simulink model "TrajectoryPlanningEmulation"  (R2018b)
settings: configuration reference "Active" (kept outside this file)
model workspace (MAT data in the model file):
  Raceline.s_m = [0 0 0 0 0 0 0 0 0 0 0 0 ... (5000 elements, 5000x1)]
  Raceline.x_m = [0 0 0 0 0 0 0 0 0 0 0 0 ... (5000 elements, 5000x1)]
  Raceline.y_m = [0 0 0 0 0 0 0 0 0 0 0 0 ... (5000 elements, 5000x1)]
  Raceline.psi_rad = [0 0 0 0 0 0 0 0 0 0 0 0 ... (5000 elements, 5000x1)]
  Raceline.kappa_radpm = [0 0 0 0 0 0 0 0 0 0 0 0 ... (5000 elements, 5000x1)]
  Raceline.vx_mps = [0 0 0 0 0 0 0 0 0 0 0 0 ... (5000 elements, 5000x1)]
  Raceline.ax_mps2 = [0 0 0 0 0 0 0 0 0 0 0 0 ... (5000 elements, 5000x1)]
  Raceline.delta_rad = [0 0 0 0 0 0 0 0 0 0 0 0 ... (5000 elements, 5000x1)]
  Raceline.F_N = [0 0 0 0 0 0 0 0 0 0 0 0 ... (5000 elements, 5000x1)]
  Raceline.ValidPointCnt = 0
  Raceline.s_m_end = 0
undefined symbols (not defined in the file): ActivateTP_PX2, P_PX2_VirtualDelay_s, tS, tSSlow, TUMHealthStatus, TUMStrategyState, TUMVehicleState
settings Model: DataDictionary=TrajectoryPlanningEmulation.sldd  ParameterArgumentNames=Raceline  OrderedModelArguments=off  Creator=wischnewski  LastModifiedBy=ge34qer

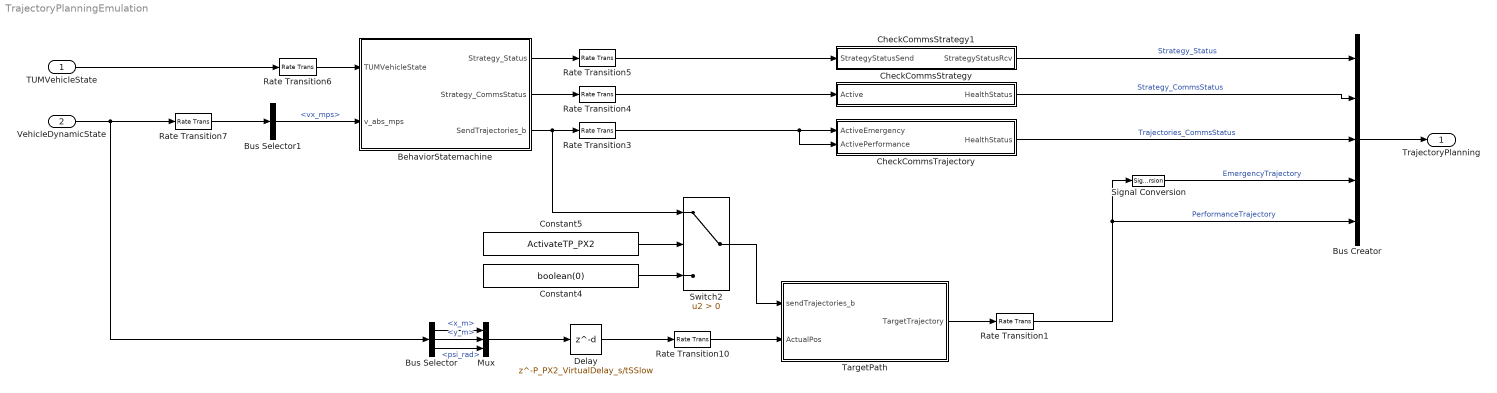
== system TrajectoryPlanningEmulation ==
  TUMVehicleState : Inport  OutDataTypeStr=Enum: TUMVehicleState  SampleTime=tS
  VehicleDynamicState : Inport  Port=2  OutDataTypeStr=Bus: VehicleDynamicState  SampleTime=tS
  BehaviorStatemachine : Subsystem  TreatAsAtomicUnit=on  SystemSampleTime=tSSlow
  Bus Creator : BusCreator  Inputs=5
  Bus Selector : BusSelector  OutputSignals=Pos.x_m,Pos.y_m,Pos.psi_rad
  Bus Selector1 : BusSelector  OutputSignals=vx_mps
  CheckCommsStrategy : Subsystem
  CheckCommsStrategy1 : Subsystem
  CheckCommsTrajectory : Subsystem
  Constant4 : Constant  Value=boolean(0)
  Constant5 : Constant  Value=ActivateTP_PX2
  Delay : Delay  DelayLength=P_PX2_VirtualDelay_s/tSSlow
  Mux : Mux  Inputs=3
  Rate Transition{1,3..4,7,10} (5 alike) : RateTransition
  Rate Transition5 : RateTransition  InitialCondition=TUMStrategyState.S_OFF
  Rate Transition6 : RateTransition  InitialCondition=TUMVehicleState.OFF
  Signal Conversion : SignalConversion  OverrideOpt=off
  Switch2 : Switch  Criteria=u2 > Threshold
  TargetPath : Subsystem  TreatAsAtomicUnit=on  SystemSampleTime=tSSlow
  TrajectoryPlanning : Outport  OutDataTypeStr=Bus: TrajectoryPlanning  SampleTime=tS  BusOutputAsStruct=on
  wires:
  Bus Creator/1 -> TrajectoryPlanning/1
  Signal Conversion/1 -> Bus Creator/4  "EmergencyTrajectory"
  VehicleDynamicState/1 -> Bus Selector/1, Rate Transition7/1
  Delay/1 -> Rate Transition10/1
  BehaviorStatemachine/1(Strategy_Status) -> Rate Transition5/1
  BehaviorStatemachine/2(Strategy_CommsStatus) -> Rate Transition4/1
  CheckCommsTrajectory/1(HealthStatus) -> Bus Creator/3  "Trajectories_CommsStatus"
  Rate Transition1/1 -> Signal Conversion/1, Bus Creator/5  "PerformanceTrajectory"
  TargetPath/1(TargetTrajectory) -> Rate Transition1/1
  CheckCommsStrategy/1(HealthStatus) -> Bus Creator/2  "Strategy_CommsStatus"
  CheckCommsStrategy1/1(StrategyStatusRcv) -> Bus Creator/1  "Strategy_Status"
  Rate Transition6/1 -> BehaviorStatemachine/1(TUMVehicleState)
  Rate Transition7/1 -> Bus Selector1/1
  Rate Transition4/1 -> CheckCommsStrategy/1(Active)
  Rate Transition5/1 -> CheckCommsStrategy1/1(StrategyStatusSend)
  Constant5/1 -> Switch2/2
  BehaviorStatemachine/3(SendTrajectories_b) -> Switch2/1, Rate Transition3/1
  Constant4/1 -> Switch2/3
  Rate Transition3/1 -> CheckCommsTrajectory/2(ActivePerformance), CheckCommsTrajectory/1(ActiveEmergency)
  Switch2/1 -> TargetPath/1(sendTrajectories_b)
  Bus Selector1/1 -> BehaviorStatemachine/2(v_abs_mps)  "<vx_mps>"
  Rate Transition10/1 -> TargetPath/2(ActualPos)
  Bus Selector/2 -> Mux/2  "<y_m>"
  Bus Selector/1 -> Mux/1  "<x_m>"
  Bus Selector/3 -> Mux/3  "<psi_rad>"
  Mux/1 -> Delay/1
  TUMVehicleState/1 -> Rate Transition6/1

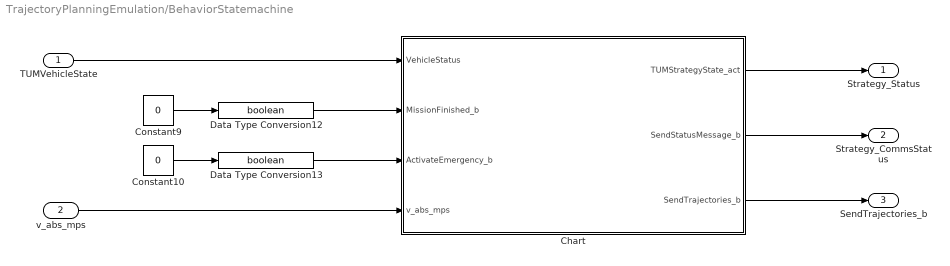
== system TrajectoryPlanningEmulation/BehaviorStatemachine ==
  TUMVehicleState : Inport  OutDataTypeStr=Enum: TUMVehicleState
  v_abs_mps : Inport  Port=2
  Chart : Stateflow chart  TreatAsAtomicUnit=on
  Constant10 : Constant  Value=0
  Constant9 : Constant  Value=0
  Data Type Conversion12 : DataTypeConversion  OutDataTypeStr=boolean
  Data Type Conversion13 : DataTypeConversion  OutDataTypeStr=boolean
  Strategy_Status : Outport
  Strategy_CommsStatus : Outport  Port=2
  SendTrajectories_b : Outport  Port=3
  wires:
  Constant10/1 -> Data Type Conversion13/1
  Data Type Conversion13/1 -> Chart/3(ActivateEmergency_b)
  v_abs_mps/1 -> Chart/4(v_abs_mps)
  Chart/3(SendTrajectories_b) -> SendTrajectories_b/1
  TUMVehicleState/1 -> Chart/1(VehicleStatus)
  Data Type Conversion12/1 -> Chart/2(MissionFinished_b)
  Constant9/1 -> Data Type Conversion12/1
  Chart/2(SendStatusMessage_b) -> Strategy_CommsStatus/1
  Chart/1(TUMStrategyState_act) -> Strategy_Status/1

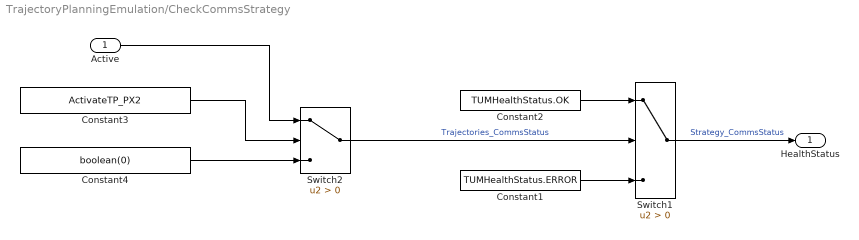
== system TrajectoryPlanningEmulation/CheckCommsStrategy ==
  Active : Inport
  Constant1 : Constant  Value=TUMHealthStatus.ERROR  OutDataTypeStr=Enum: TUMHealthStatus
  Constant2 : Constant  Value=TUMHealthStatus.OK  OutDataTypeStr=Enum: TUMHealthStatus
  Constant3 : Constant  Value=ActivateTP_PX2
  Constant4 : Constant  Value=boolean(0)
  Switch1 : Switch  Criteria=u2 > Threshold
  Switch2 : Switch  Criteria=u2 > Threshold
  HealthStatus : Outport
  wires:
  Constant2/1 -> Switch1/1
  Switch1/1 -> HealthStatus/1  "Strategy_CommsStatus"
  Constant1/1 -> Switch1/3
  Constant3/1 -> Switch2/2
  Active/1 -> Switch2/1
  Constant4/1 -> Switch2/3
  Switch2/1 -> Switch1/2  "Trajectories_CommsStatus"

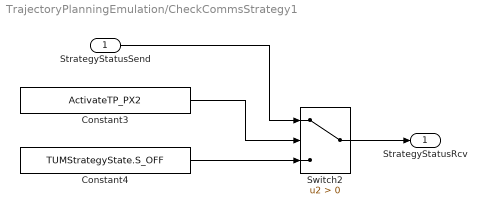
== system TrajectoryPlanningEmulation/CheckCommsStrategy1 ==
  StrategyStatusSend : Inport
  Constant3 : Constant  Value=ActivateTP_PX2
  Constant4 : Constant  Value=TUMStrategyState.S_OFF
  Switch2 : Switch  Criteria=u2 > Threshold
  StrategyStatusRcv : Outport
  wires:
  Constant3/1 -> Switch2/2
  StrategyStatusSend/1 -> Switch2/1
  Constant4/1 -> Switch2/3
  Switch2/1 -> StrategyStatusRcv/1

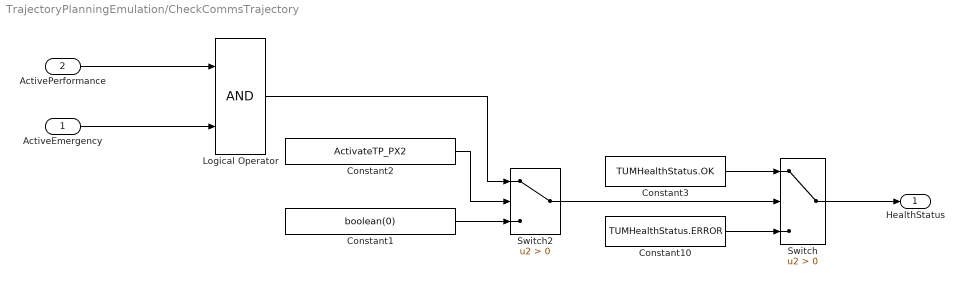
== system TrajectoryPlanningEmulation/CheckCommsTrajectory ==
  ActiveEmergency : Inport
  ActivePerformance : Inport  Port=2
  Constant1 : Constant  Value=boolean(0)
  Constant10 : Constant  Value=TUMHealthStatus.ERROR  OutDataTypeStr=Enum: TUMHealthStatus
  Constant2 : Constant  Value=ActivateTP_PX2
  Constant3 : Constant  Value=TUMHealthStatus.OK  OutDataTypeStr=Enum: TUMHealthStatus
  Logical Operator : Logic  AllPortsSameDT=off  OutDataTypeStr=boolean
  Switch : Switch  Criteria=u2 > Threshold
  Switch2 : Switch  Criteria=u2 > Threshold
  HealthStatus : Outport
  wires:
  Constant10/1 -> Switch/3
  Switch2/1 -> Switch/2
  Constant3/1 -> Switch/1
  Switch/1 -> HealthStatus/1
  Constant2/1 -> Switch2/2
  Logical Operator/1 -> Switch2/1
  Constant1/1 -> Switch2/3
  ActivePerformance/1 -> Logical Operator/1
  ActiveEmergency/1 -> Logical Operator/2

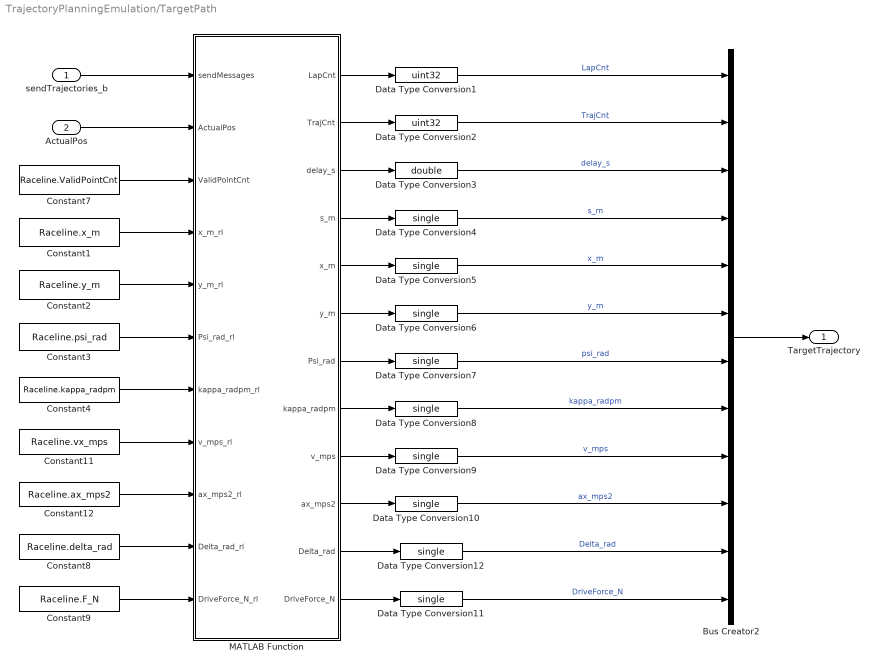
== system TrajectoryPlanningEmulation/TargetPath ==
  sendTrajectories_b : Inport
  ActualPos : Inport  Port=2  PortDimensions=3
  Bus Creator2 : BusCreator  Inputs=12  OutDataTypeStr=Bus: Trajectory
      settings: InheritFromInputs=off
  Constant1 : Constant  Value=Raceline.x_m
  Constant11 : Constant  Value=Raceline.vx_mps
  Constant12 : Constant  Value=Raceline.ax_mps2
  Constant2 : Constant  Value=Raceline.y_m
  Constant3 : Constant  Value=Raceline.psi_rad
  Constant4 : Constant  Value=Raceline.kappa_radpm
  Constant7 : Constant  Value=Raceline.ValidPointCnt
  Constant8 : Constant  Value=Raceline.delta_rad
  Constant9 : Constant  Value=Raceline.F_N
  Data Type Conversion1 : DataTypeConversion  OutDataTypeStr=uint32
  Data Type Conversion{4..12} (9 alike) : DataTypeConversion  OutDataTypeStr=single
  Data Type Conversion2 : DataTypeConversion  OutDataTypeStr=uint32
  Data Type Conversion3 : DataTypeConversion  OutDataTypeStr=double
  MATLAB Function : MATLAB Function  TreatAsAtomicUnit=on
  TargetTrajectory : Outport  OutDataTypeStr=Bus: Trajectory
  wires:
  MATLAB Function/1(LapCnt) -> Data Type Conversion1/1
  Data Type Conversion4/1 -> Bus Creator2/4  "s_m"
  Data Type Conversion5/1 -> Bus Creator2/5  "x_m"
  Data Type Conversion6/1 -> Bus Creator2/6  "y_m"
  Data Type Conversion7/1 -> Bus Creator2/7  "psi_rad"
  Data Type Conversion8/1 -> Bus Creator2/8  "kappa_radpm"
  Data Type Conversion9/1 -> Bus Creator2/9  "v_mps"
  Data Type Conversion10/1 -> Bus Creator2/10  "ax_mps2"
  MATLAB Function/4(s_m) -> Data Type Conversion4/1
  MATLAB Function/5(x_m) -> Data Type Conversion5/1
  MATLAB Function/6(y_m) -> Data Type Conversion6/1
  MATLAB Function/7(Psi_rad) -> Data Type Conversion7/1
  MATLAB Function/8(kappa_radpm) -> Data Type Conversion8/1
  MATLAB Function/9(v_mps) -> Data Type Conversion9/1
  MATLAB Function/10(ax_mps2) -> Data Type Conversion10/1
  Data Type Conversion1/1 -> Bus Creator2/1  "LapCnt"
  Data Type Conversion2/1 -> Bus Creator2/2  "TrajCnt"
  Constant1/1 -> MATLAB Function/4(x_m_rl)
  Constant2/1 -> MATLAB Function/5(y_m_rl)
  Constant3/1 -> MATLAB Function/6(Psi_rad_rl)
  Constant4/1 -> MATLAB Function/7(kappa_radpm_rl)
  MATLAB Function/2(TrajCnt) -> Data Type Conversion2/1
  Constant7/1 -> MATLAB Function/3(ValidPointCnt)
  Bus Creator2/1 -> TargetTrajectory/1
  ActualPos/1 -> MATLAB Function/2(ActualPos)
  Data Type Conversion3/1 -> Bus Creator2/3  "delay_s"
  sendTrajectories_b/1 -> MATLAB Function/1(sendMessages)
  MATLAB Function/3(delay_s) -> Data Type Conversion3/1
  Data Type Conversion12/1 -> Bus Creator2/11  "Delta_rad"
  Data Type Conversion11/1 -> Bus Creator2/12  "DriveForce_N"
  MATLAB Function/11(Delta_rad) -> Data Type Conversion12/1
  MATLAB Function/12(DriveForce_N) -> Data Type Conversion11/1
  Constant8/1 -> MATLAB Function/10(Delta_rad_rl)
  Constant9/1 -> MATLAB Function/11(DriveForce_N_rl)
  Constant11/1 -> MATLAB Function/8(v_mps_rl)
  Constant12/1 -> MATLAB Function/9(ax_mps2_rl)

== matlab function TrajectoryPlanningEmulation/TargetPath/MATLAB Function ==
  data: sendMessages input; ActualPos input; ValidPointCnt input; LapCnt output size=1; x_m_rl input; y_m_rl input; Psi_rad_rl input; kappa_radpm_rl input; v_mps_rl input; ax_mps2_rl input; TrajCnt output size=1; delay_s output; s_m output size=50; x_m output size=50; y_m output size=50; Psi_rad output size=50; kappa_radpm output size=50; v_mps output size=50; ax_mps2 output size=50; Delta_rad output; DriveForce_N output; Delta_rad_rl input; DriveForce_N_rl input
function [LapCnt, TrajCnt, delay_s, s_m, x_m, y_m, Psi_rad, kappa_radpm, v_mps, ax_mps2, Delta_rad, DriveForce_N] =...
  fcn(sendMessages, ActualPos, ValidPointCnt, x_m_rl, y_m_rl, Psi_rad_rl, kappa_radpm_rl, v_mps_rl, ax_mps2_rl, Delta_rad_rl, DriveForce_N_rl)
% function wrapper for cutLocalTrajectoryFromRaceline
[LapCnt, TrajCnt, delay_s, s_m, x_m, y_m, Psi_rad, kappa_radpm, v_mps, ax_mps2, Delta_rad, DriveForce_N] =...
  cutLocalTrajectoryFromRaceline(sendMessages, ActualPos, ValidPointCnt, x_m_rl, y_m_rl, Psi_rad_rl, kappa_radpm_rl, v_mps_rl, ax_mps2_rl, Delta_rad_rl, DriveForce_N_rl);
end

== stateflow chart TrajectoryPlanningEmulation/BehaviorStatemachine/Chart ==
  state StartupStrategy
    entry: TUMStrategyState_act = ...
    TUMStrategyState.S_STARTUP;
  state SendStatusMessage
    entry: SendStatusMessage_b = true;
    exit: SendStatusMessage_b = false;
    state Idle
      entry: TUMStrategyState_act = ...
      TUMStrategyState.S_STANDSTILL;
    state Idle1
      entry: TUMStrategyState_act = ...
      TUMStrategyState.S_STANDSTILL_TRAJSEND;
      entry:  SendTrajectories_b = true;
    state DRIVING
      state Driving
        entry: TUMStrategyState_act = ...
        TUMStrategyState.S_DRIVING_NORMAL;
      state Brake2Stop
        entry: TUMStrategyState_act = ...
        TUMStrategyState.S_DRIVING_BRAKE2STOP;
      state Emergency
        entry: TUMStrategyState_act =...
        TUMStrategyState.S_DRIVING_EMERGENCY;
      Driving -> Brake2Stop [order 1] : [MissionFinished_b]
      Driving -> Emergency [order 2] : [ActivateEmergency_b]
    (default) -> Idle
    Idle -> Idle1 : [int16(VehicleStatus)  >= 22]
    Idle1 -> Driving : [VehicleStatus == TUMVehicleState.DRIVING]
  (default) -> StartupStrategy
  StartupStrategy -> SendStatusMessage : after(5, sec)
  data: TUMStrategyState_act output; SendStatusMessage_b output boolean =false; VehicleStatus input Enum: TUMVehicleState; SendTrajectories_b output boolean; MissionFinished_b input boolean; ActivateEmergency_b input boolean; P_PX2_EnterIdle_mps parameter; v_abs_mps input
